simulink model "PMDC_K11"  (R2025a)
settings: Solver=VariableStepAuto  StartTime=0.0  StopTime=50e-3  MaxStep=329e-6/25  RelTol=1e-3
settings Model: Creator=Szalay  LastModifiedBy=Szalay

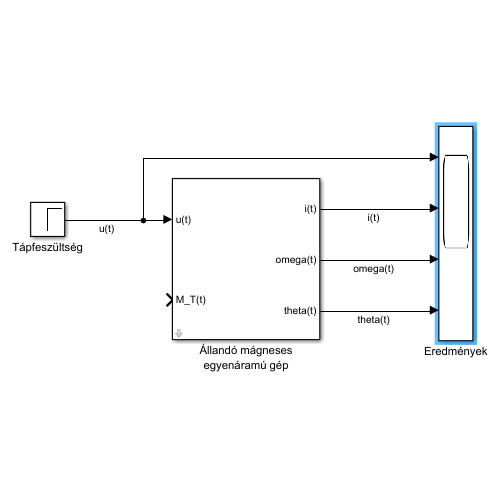
[thumbnail: Simulink's stored preview of the top-level diagram]
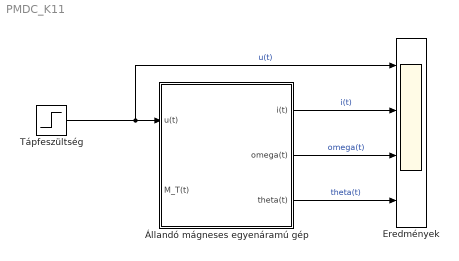
== system PMDC_K11 ==
  Eredmények : Scope  NumInputPorts=4
      settings: ActiveDisplayString=4  ActiveDisplayYMinimum=-4.8967215005520881  ActiveDisplayYMaximum=44.0704935049688
  Tápfeszültség : Step  Time=1e-3  After=12  SampleTime=0
  Állandó mágneses egyenáramú gép : Subsystem  mask(Állandó mágneses egyenáramú gép){R=79e-3, L=26e-6, k_E=13.7e-3, k_T=13.7e-3, J=99.5e-7, B=5.15e-6, i_0=0, omega_0=0, theta_0=0}
      mask prompts: R "Armatúra ellenállás"; L "Armatúra induktivitás"; k_E "Feszültségállandó"; k_T "Nyomatékállandó"; J "Tehetetlenségi nyomaték"; B "Forgási súrlódási együttható"; i_0 "Kezdeti áramerősség"; omega_0 "Kezdeti szögsebesség"; theta_0 "Kezdeti szöghelyzet"
      mask help: Az állandó mágneses egyenáramú gép modellje a Maxon DCX 35L típus alapján paraméterezve.
      mask DialogControl Container3 Prompt: Modellparaméterek
      mask DialogControl Container5 Prompt: Villamos áramköri rész
      mask DialogControl Container6 Prompt: Mágnesköri gépállandók
      mask DialogControl Container7 Prompt: Forgó részrendszer
      mask DialogControl Container4 Prompt: Kezdeti értékek
      mask DialogControl Container8 Prompt: Villamos áramköri rész
      mask DialogControl Container9 Prompt: Forgó részrendszer
  wires:
  Tápfeszültség/1 -> Eredmények/1, Állandó mágneses egyenáramú gép/1(u(t))  "u(t)"
  Állandó mágneses egyenáramú gép/1(i(t)) -> Eredmények/2  "i(t)"
  Állandó mágneses egyenáramú gép/2(omega(t)) -> Eredmények/3  "omega(t)"
  Állandó mágneses egyenáramú gép/3(theta(t)) -> Eredmények/4  "theta(t)"

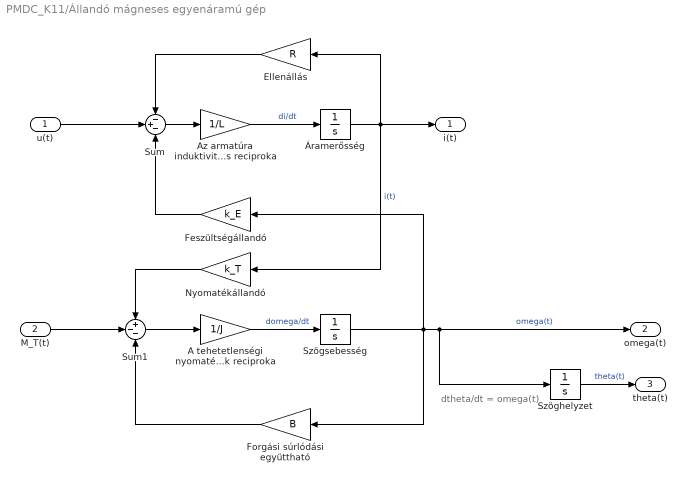
== system PMDC_K11/Állandó mágneses egyenáramú gép ==
  note: dtheta/dt = omega(t)
  u(t) : Inport
  M_T(t) : Inport  Port=2
  A tehetetlenségi nyomaték reciproka : Gain  Gain=1/J
  Az armatúra induktivitás reciproka : Gain  Gain=1/L
  Ellenállás : Gain  Gain=R
  Feszültségállandó : Gain  Gain=k_E
  Forgási súrlódási együttható : Gain  Gain=B
  Nyomatékállandó : Gain  Gain=k_T
  Sum : Sum  Inputs=-+-
  Sum1 : Sum  Inputs=+--
  Szöghelyzet : Integrator
  Szögsebesség : Integrator
  Áramerősség : Integrator
  i(t) : Outport
  omega(t) : Outport  Port=2
  theta(t) : Outport  Port=3
  wires:
  Szögsebesség/1 -> omega(t)/1, Szöghelyzet/1, Feszültségállandó/1, Forgási súrlódási együttható/1  "omega(t)"
  Áramerősség/1 -> i(t)/1, Nyomatékállandó/1, Ellenállás/1  "i(t)"
  Sum1/1 -> A tehetetlenségi nyomaték reciproka/1
  Az armatúra induktivitás reciproka/1 -> Áramerősség/1  "di/dt"
  Forgási súrlódási együttható/1 -> Sum1/3
  A tehetetlenségi nyomaték reciproka/1 -> Szögsebesség/1  "domega/dt"
  Sum/1 -> Az armatúra induktivitás reciproka/1
  Feszültségállandó/1 -> Sum/3
  Nyomatékállandó/1 -> Sum1/1
  M_T(t)/1 -> Sum1/2
  Ellenállás/1 -> Sum/1
  u(t)/1 -> Sum/2
  Szöghelyzet/1 -> theta(t)/1  "theta(t)"
